simulink model "PIDRelaylab"  (Simulink 7.0)
settings: Solver=FixedStepDiscrete  StartTime=0.0  StopTime=inf  FixedStep=0.5  RelTol=1e-3
libraries: SuperLogic x3, simulink x1, RT x1
settings Model: Creator=ugur  LastModifiedBy=xx  SimulationMode=accelerator
settings DataIOCC: LimitDataPoints=off
settings OptimizationCC: InlineInvariantSignals=on
settings DebuggingCC: SaveWithParameterizedLinksMsg=none  SignalResolutionControl=TryResolveAllWithWarning  MultiTaskDSMMsg=warning  MultiTaskCondExecSysMsg=none  StrictBusMsg=None
settings RTWCC: IncludeERTFirstTime=on
settings GRTTargetCC: TargetFcnLib=ansi_tfl_tmw.mat

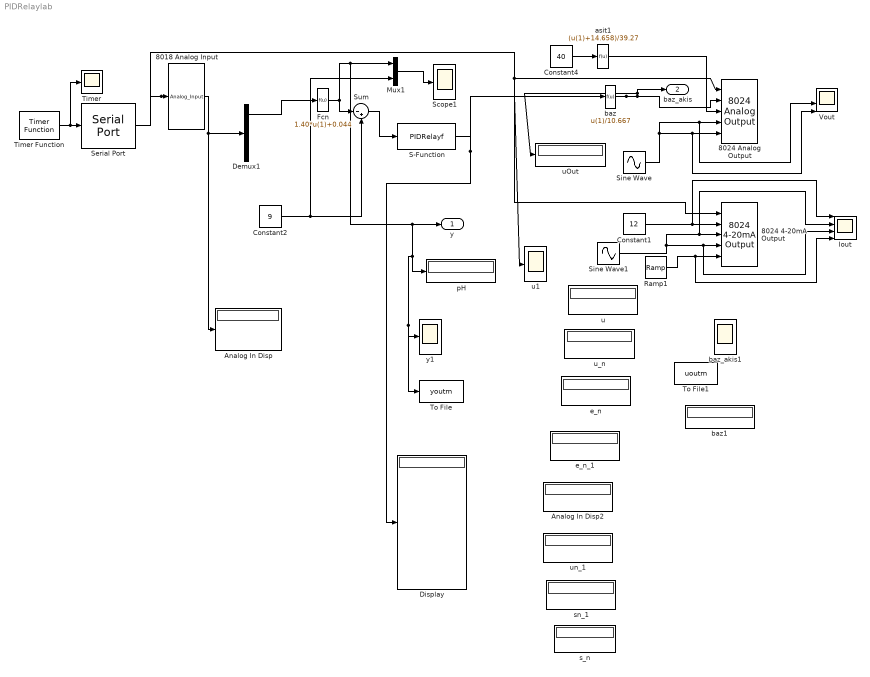
== system PIDRelaylab ==
  8018 Analog Input : S-Function  FunctionName=Analog_Input  Parameters=AC1, AC2, AC3, AC4, AC5, AC6, AC7, AC8  mask(S function: Analog Input){AC1=off, AC2=on, AC3=off, AC4=off, AC5=on, AC6=on, AC7=off, AC8=off}
      mask prompts: AC1 "Analog Channel 1"; AC2 "Analog Channel 2"; AC3 "Analog Channel 3"; AC4 "Analog Channel 4"; AC5 "Analog Channel 5"; AC6 "Analog Channel 6"; AC7 "Analog Channel 7"; AC8 "Analog Channel 8"
      mask help:
      | This M-file reads the analog input channels from the SL 8018 with 8520
      | The first input is the Com_port number from Serial Port Block.
      mask Display: image(imread('8018.jpg'))
  8024 4-20mA Output : SuperLogic/8024 4-20mA Output  SystemSampleTime=-1  OC1=on  OC2=on  OC3=on  OC4=on
  8024 Analog Output : SuperLogic/8024 Analog Output  SystemSampleTime=-1  OC1=on  OC2=on  OC3=on  OC4=on
  Analog In Disp : Display
  Analog In Disp2 : Display
      settings: Decimation=2
  Constant1 : Constant  Value=12  OutDataType=sfix(16)  OutScaling=2^0
  Constant2 : Constant  Value=9  OutDataType=sfix(16)  OutScaling=2^0
  Constant4 : Constant  Value=40  OutDataType=sfix(16)  OutScaling=2^0
  Demux1 : Demux  Outputs=3
  Display : Display
  Fcn : Fcn  Expr=1.40*u(1)+0.044
  Iout : Scope  NumInputPorts=4
      settings: TimeRange=10  YMin=0~0~0~0  YMax=24~24~24~24  SaveName=ScopeData3  SampleInput=on
  Mux1 : Mux  Inputs=2
  Ramp1 : simulink/Sources/Ramp  SystemSampleTime=-1  slope=0.5  start=0  X0=4
  S-Function : S-Function  FunctionName=PIDRelayf
  Scope1 : Scope
      settings: TimeRange=10000  YMin=0  YMax=12  SaveName=ScopeData4  SampleInput=on
  Serial Port : SuperLogic/Serial Port  PORT_NAME=COM1  PORT_BRATE=19200
  Sine Wave : Sin  Amplitude=4  Bias=6  Frequency=pi/5  SampleTime=0
  Sine Wave1 : Sin  Amplitude=8  Bias=12  Frequency=pi/5  SampleTime=0
  Sum : Sum  Inputs=|-+  OutDataType=sfix(16)  OutScaling=2^0
  Timer : Scope
      settings: TimeRange=30  YMin=0  YMax=500
  Timer Function : RT/Timer Function  Priority=245354192  step=500  tmrpriority=HIGH  ThPriority=NORMAL
  To File : ToFile  Filename=youtm
  To File1 : ToFile  Filename=uoutm
  Vout : Scope  NumInputPorts=4
      settings: TimeRange=10  YMin=0~0~0~0  YMax=10~10~10~10  SaveName=ScopeData2  SampleInput=on
  asit1 : Fcn  Expr=(u(1)+14.658)/39.27
  baz : Fcn  Expr=u(1)/10.667
  baz1 : Display
  baz_akis1 : Scope
      settings: TimeRange=5000  YMin=10  YMax=20  SaveName=ScopeData5  SampleInput=on
  e_n : Display
      settings: Decimation=2
  e_n_1 : Display
      settings: Decimation=2
  pH : Display
  s_n : Display
      settings: Decimation=2
  sn_1 : Display
      settings: Decimation=2
  u : Display
      settings: Decimation=2
  u1 : Scope
      settings: TimeRange=5000  YMin=2.5  YMax=11  SaveName=ScopeData6  SampleInput=on
  uOut : Display
  u_n : Display
      settings: Decimation=2
  un_1 : Display
      settings: Decimation=2
  y1 : Scope
      settings: TimeRange=5000  YMin=6.5  YMax=10  SampleInput=on
  y : Outport  OutDataType=sfix(16)  OutScaling=2^0
  baz_akis : Outport  Port=2  OutDataType=sfix(16)  OutScaling=2^0
  wires:
  Serial Port/1 -> 8018 Analog Input/1, 8024 4-20mA Output/1, 8024 Analog Output/1
  Timer Function/1 -> Serial Port/1, Timer/1
  8018 Analog Input/1 -> Analog In Disp/1, Demux1/1
  Constant1/1 -> Iout/1, 8024 4-20mA Output/2
  Ramp1/1 -> 8024 4-20mA Output/5, Iout/4
  Sine Wave/1 -> 8024 Analog Output/4, Vout/3, 8024 Analog Output/5, Vout/4
  Sine Wave1/1 -> 8024 4-20mA Output/3, Iout/2, 8024 4-20mA Output/4, Iout/3
  Constant2/1 -> Sum/2, Mux1/2
  Fcn/1 -> Sum/1, Mux1/1, y/1, pH/1, y1/1, To File/1
  S-Function/1 -> Display/1, baz/1
  Mux1/1 -> Scope1/1
  Demux1/1 -> Fcn/1
  baz/1 -> 8024 Analog Output/2, baz_akis/1, uOut/1, u1/1
  asit1/1 -> 8024 Analog Output/3
  Constant4/1 -> asit1/1
  Sum/1 -> S-Function/1
